simulink model "tanque"  (R2024a)
settings: Solver=VariableStepAuto  StartTime=0.0  StopTime=500  RelTol=1e-3

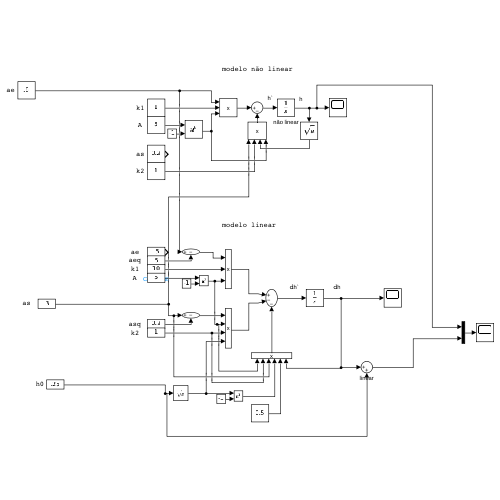
[thumbnail: Simulink's stored preview of the top-level diagram]
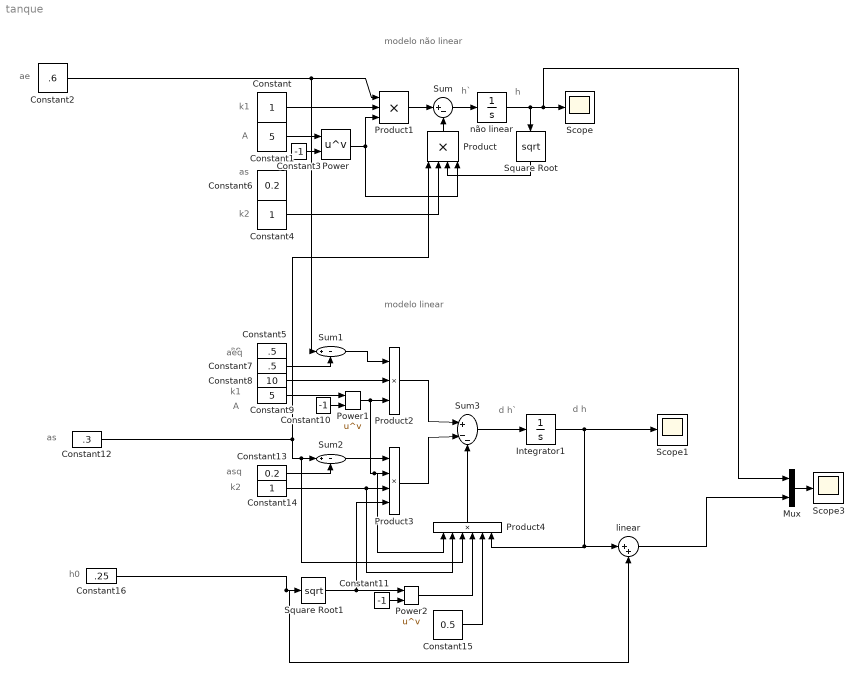
== system tanque ==
  note: ae
  note: A
  note: k1
  note: h`
  note: k2
  note: as
  note: h
  note: modelo não linear
  note: ae
  note: aeq
  note: k1
  note: A
  note: k2
  note: as
  note: asq
  note: h0
  note: d h`
  note: d h
  note: modelo linear
  Constant : Constant
  Constant1 : Constant  Value=5
  Constant10 : Constant  Value=-1
  Constant11 : Constant  Value=-1
  Constant12 : Constant  Value=.3
  Constant13 : Constant  Value=0.2
  Constant14 : Constant
  Constant15 : Constant  Value=0.5
  Constant16 : Constant  Value=.25
  Constant2 : Constant  Value=.6
  Constant3 : Constant  Value=-1
  Constant4 : Constant
  Constant5 : Constant  Value=.5
  Constant6 : Constant  Value=0.2
  Constant7 : Constant  Value=.5
  Constant8 : Constant  Value=10
  Constant9 : Constant  Value=5
  Integrator1 : Integrator
  Mux : Mux  Inputs=2
  Power : Math  Operator=pow
  Power1 : Math  Operator=pow
  Power2 : Math  Operator=pow
  Product : Product  Inputs=4
  Product1 : Product  Inputs=3
  Product2 : Product  Inputs=3
  Product3 : Product  Inputs=4
  Product4 : Product  Inputs=6
  Scope : Scope
  Scope1 : Scope
  Scope3 : Scope
  Square Root : Sqrt
  Square Root1 : Sqrt
  Sum : Sum  Inputs=|+-
  Sum1 : Sum  Inputs=|+-
  Sum2 : Sum  Inputs=|+-
  Sum3 : Sum  Inputs=|+--
  linear : Sum  Inputs=|++
  não linear : Integrator  InitialCondition=.25
  wires:
  Constant3/1 -> Power/2
  Constant1/1 -> Power/1
  Constant/1 -> Product1/2
  Power/1 -> Product/4, Product1/3
  Constant2/1 -> Sum1/1, Product1/1
  Product1/1 -> Sum/1
  Sum/1 -> não linear/1
  Product/1 -> Sum/2
  Constant4/1 -> Product/2
  Square Root/1 -> Product/3
  não linear/1 -> Mux/1, Scope/1, Square Root/1
  Constant7/1 -> Sum1/2
  Constant10/1 -> Power1/2
  Constant9/1 -> Power1/1
  Constant8/1 -> Product2/2
  Sum1/1 -> Product2/1
  Constant12/1 -> Product4/3, Sum2/1, Product/1
  Constant13/1 -> Sum2/2
  Sum2/1 -> Product3/1
  Constant14/1 -> Product3/3, Product4/2
  Square Root1/1 -> Power2/1, Product3/4
  Constant16/1 -> linear/2, Square Root1/1
  Power1/1 -> Product3/2, Product4/1, Product2/3
  Product4/1 -> Sum3/3
  Product3/1 -> Sum3/2
  Product2/1 -> Sum3/1
  Sum3/1 -> Integrator1/1
  Integrator1/1 -> Scope1/1, linear/1, Product4/6
  Constant11/1 -> Power2/2
  Power2/1 -> Product4/4
  Constant15/1 -> Product4/5
  linear/1 -> Mux/2
  Mux/1 -> Scope3/1
